simulink model "homework3_question2e_Sim"  (R2024a)
settings: Solver=VariableStepAuto  StartTime=0.0  StopTime=10.0  RelTol=1e-3
libraries: simulink x1
settings Model: Creator=mamad  LastModifiedBy=mamad

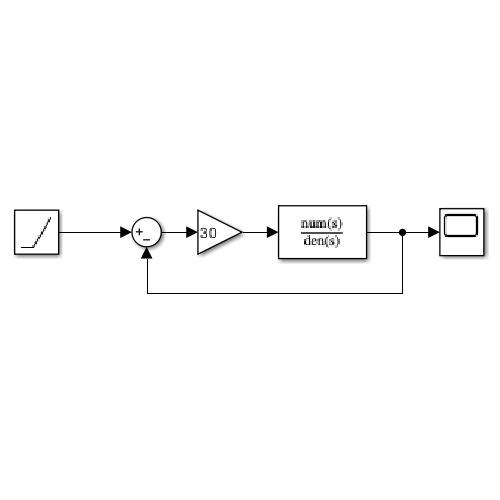
[thumbnail: Simulink's stored preview of the top-level diagram]
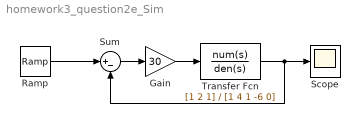
== system homework3_question2e_Sim ==
  Gain : Gain  Gain=30
  Ramp : simulink/Sources/Ramp  slope=1  start=0  InitialOutput=0
  Scope : Scope
  Sum : Sum  Inputs=|+-
  Transfer Fcn : TransferFcn  Numerator=[1 2 1]  Denominator=[1 4 1 -6 0]
  wires:
  Ramp/1 -> Sum/1
  Sum/1 -> Gain/1
  Gain/1 -> Transfer Fcn/1
  Transfer Fcn/1 -> Scope/1, Sum/2
